simulink library "qss_tb_library_aalto"  (Simulink 8.3)
settings: Solver=ode45  SolverMode=SingleTasking  StartTime=0.0  StopTime=1220  RelTol=1e-3
undefined symbols (not defined in the file): c_BT_E1, c_BT_E2, c_BT_E3, c_BT_E4, c_BT_L1, c_BT_L2, c_BT_L3, c_BT_L4, cap_BT, cc_done, delta_h_C_air, DiscIntNeverNeededParam, dw_GG_c, eff_FC_max, eta_EG_map, eta_EM_map, g, h, H_o_m, H_u, I_BT_max, i_FC_in, i_FC_max, k1, k2, k3, k4, k_cs, M_air, manual_gearbox, P_CVT_opt, power_max, Q_BT_0, Q_BT_IC, Q_BT_min, Q_SC_IC, r_wheel, rchg_map_BT, rdis_map_BT, rho, rho_f, soc_map_BT, t_c, T_CE_max, T_EG_c, T_EG_max, T_EM_max, T_z, U_BT_0, V, V_CE_map, V_FC_out, voc_map_BT, w_CE_max, w_CE_upper, w_CVT_opt, w_EG_row, w_EG_upper, w_EM_row, w_EM_upper ... (+1)
libraries: simulink x4
(part 2 of 4)

== system qss_tb_library_aalto/Energy Buffer/Supercapacitor v2 ==
  P_SC : Inport
  Fcn : Fcn  Expr=(-u[2]/C_SC+sqrt(u[2]^2/C_SC^2-4*R_SC*u[1]))/(2*R_SC)
  Gain : Gain  Gain=1/C_SC  SaturateOnIntegerOverflow=on  OutDataTypeStr=Inherit: Same as input  ParamDataTypeStr=Inherit: Same as input
  Gain1 : Gain  Gain=h  SaturateOnIntegerOverflow=on  OutDataTypeStr=Inherit: Same as input  ParamDataTypeStr=Inherit: Same as input
  Mux : Mux  Inputs=2
  SC charge : UnitDelay  InitialCondition=Q_SC_IC  SampleTime=h
  Sum3 : Sum  SaturateOnIntegerOverflow=on  InputSameDT=on  OutDataTypeStr=Inherit: Same as first input
  Supervision supercap : Subsystem
  To Workspace1 : ToWorkspace  VariableName=I_SC  SampleTime=1
  To Workspace2 : ToWorkspace  VariableName=U_SC  SampleTime=1
  To Workspace3 : ToWorkspace  VariableName=Q_SC  SampleTime=1
  To Workspace4 : ToWorkspace  VariableName=P_SC  SampleTime=1
  U_SC : Outport  InitialOutput=0
  wires:
  Gain1/1 -> Sum3/1
  Mux/1 -> Fcn/1
  Sum3/1 -> SC charge/1
  SC charge/1 -> Sum3/2, Gain/1, Mux/2, Supervision supercap/1(Q_SC), To Workspace3/1
  Fcn/1 -> Gain1/1, To Workspace1/1
  Gain/1 -> U_SC/1, To Workspace2/1
  P_SC/1 -> To Workspace4/1, Mux/1, Supervision supercap/2(P_SC)

== system qss_tb_library_aalto/Energy Buffer/Supercapacitor v3 ==
  P_SC : Inport
  Fcn : Fcn  Expr=(-u[2]/C_SC+sqrt(u[2]^2/C_SC^2-4*R_SC*u[1]))/(2*R_SC)
  Gain : Gain  Gain=1/C_SC  SaturateOnIntegerOverflow=on  OutDataTypeStr=Inherit: Same as input  ParamDataTypeStr=Inherit: Same as input
  Gain1 : Gain  Gain=h  SaturateOnIntegerOverflow=on  OutDataTypeStr=Inherit: Same as input  ParamDataTypeStr=Inherit: Same as input
  Mux : Mux  Inputs=2
  SC charge : UnitDelay  InitialCondition=Q_SC_IC  SampleTime=h
  Sum3 : Sum  SaturateOnIntegerOverflow=on  InputSameDT=on  OutDataTypeStr=Inherit: Same as first input
  Supervision supercap : Subsystem
  To Workspace1 : ToWorkspace  VariableName=I_SC  SampleTime=1
  To Workspace2 : ToWorkspace  VariableName=U_SC  SampleTime=1
  To Workspace3 : ToWorkspace  VariableName=Q_SC  SampleTime=1
  To Workspace4 : ToWorkspace  VariableName=P_SC  SampleTime=1
  U_SC : Outport  InitialOutput=0
  wires:
  P_SC/1 -> Supervision supercap/2(P_SC), Mux/1, To Workspace4/1
  Gain/1 -> To Workspace2/1, U_SC/1
  Fcn/1 -> To Workspace1/1, Gain1/1
  SC charge/1 -> To Workspace3/1, Supervision supercap/1(Q_SC), Mux/2, Gain/1, Sum3/2
  Sum3/1 -> SC charge/1
  Mux/1 -> Fcn/1
  Gain1/1 -> Sum3/1

== system qss_tb_library_aalto/Energy Converter/Combustion Engine (Willans-approximation) ==
  w_gear : Inport
  dw_gear : Inport  Port=2
  T_gear : Inport  Port=3
  Constant1 : Constant  Value=P_aux
  Detect fuel cutoff : Subsystem
  Detect idle : Subsystem
  Engine efficiency : Subsystem
  Engine inertia : Gain  Gain=theta_CE  SaturateOnIntegerOverflow=on  OutDataTypeStr=Inherit: Same as input  ParamDataTypeStr=Inherit: Same as input
  Lower limit (fuel cutoff) : Saturate  UpperLimit=inf  LowerLimit=T_CE_cutoff
  Lower limit (speed at idle) : Saturate  UpperLimit=inf  LowerLimit=w_CE_idle
  Product : Product  Inputs=**/  SaturateOnIntegerOverflow=on  RndMeth=Zero  InputSameDT=on  OutDataTypeStr=Inherit: Same as first input
  To Workspace3 : ToWorkspace  VariableName=T_CE  SampleTime=-1
  To Workspace4 : ToWorkspace  VariableName=w_CE  SampleTime=-1
  To Workspace5 : ToWorkspace  VariableName=P_CE  SampleTime=-1
  Total power : Sum  SaturateOnIntegerOverflow=on  InputSameDT=on  OutDataTypeStr=Inherit: Same as first input
  Total torque : Sum  SaturateOnIntegerOverflow=on  InputSameDT=on  OutDataTypeStr=Inherit: Same as first input
  P_CE : Outport  InitialOutput=0
  wires:
  Engine efficiency/1(eta_CE) -> Product/3
  T_gear/1 -> Total torque/1
  dw_gear/1 -> Engine inertia/1
  Total torque/1 -> Lower limit (fuel cutoff)/1
  Engine inertia/1 -> Total torque/2
  Lower limit (fuel cutoff)/1 -> Detect idle/3(T_CE), Detect fuel cutoff/2(T_CE), Engine efficiency/2(T_CE), Product/2, To Workspace3/1
  Lower limit (speed at idle)/1 -> To Workspace4/1, Engine efficiency/1(w_CE), Detect idle/2(w_CE), Product/1
  w_gear/1 -> Lower limit (speed at idle)/1
  Product/1 -> Detect idle/1(P_CE_fuel)
  Detect idle/1(P_CE) -> Detect fuel cutoff/1(P_CE_fuel)
  Detect fuel cutoff/1(P_CE) -> Total power/1
  Total power/1 -> P_CE/1, To Workspace5/1
  Constant1/1 -> Total power/2

== system qss_tb_library_aalto/Energy Converter/Combustion Engine (consumption map) ==
  w_gear : Inport
  dw_gear : Inport  Port=2
  T_gear : Inport  Port=3
  Constant1 : Constant  Value=P_aux
  Detect fuel cutoff : Subsystem
  Detect idle : Subsystem
  Detect overload and overspeed : Subsystem
  "Engine consumption map V = f(w, T) [kg/s]" : Lookup2D  RowIndex=w_CE_row  ColumnIndex=T_CE_col  Table=V_CE_map
  Engine inertia : Gain  Gain=theta_CE  SaturateOnIntegerOverflow=on  OutDataTypeStr=Inherit: Same as input  ParamDataTypeStr=Inherit: Same as input
  Fuel lower heating value : Gain  Gain=H_u  SaturateOnIntegerOverflow=on  OutDataTypeStr=Inherit: Same as input  ParamDataTypeStr=Inherit: Same as input
  Lower limit (fuel cutoff) : Saturate  UpperLimit=inf  LowerLimit=T_CE_cutoff
  Lower limit (speed at idle) : Saturate  UpperLimit=inf  LowerLimit=w_CE_idle
  To Workspace3 : ToWorkspace  VariableName=T_CE  SampleTime=-1
  To Workspace4 : ToWorkspace  VariableName=w_CE  SampleTime=-1
  To Workspace5 : ToWorkspace  VariableName=P_CE  SampleTime=-1
  Total power : Sum  SaturateOnIntegerOverflow=on  InputSameDT=on  OutDataTypeStr=Inherit: Same as first input
  Total torque : Sum  SaturateOnIntegerOverflow=on  InputSameDT=on  OutDataTypeStr=Inherit: Same as first input
  P_CE : Outport  InitialOutput=0
  wires:
  T_gear/1 -> Total torque/1
  dw_gear/1 -> Engine inertia/1
  Total torque/1 -> Lower limit (fuel cutoff)/1
  Engine inertia/1 -> Total torque/2
  Lower limit (speed at idle)/1 -> Detect overload and overspeed/1(w_CE), Detect idle/2(w_CE), "Engine consumption map V = f(w, T) [kg/s]"/1, To Workspace4/1
  w_gear/1 -> Lower limit (speed at idle)/1
  Fuel lower heating value/1 -> Detect idle/1(P_CE_fuel)
  Detect idle/1(P_CE) -> Detect fuel cutoff/1(P_CE_fuel)
  "Engine consumption map V = f(w, T) [kg/s]"/1 -> Fuel lower heating value/1
  Detect fuel cutoff/1(P_CE) -> Total power/1
  Total power/1 -> P_CE/1, To Workspace5/1
  Constant1/1 -> Total power/2
  Lower limit (fuel cutoff)/1 -> Detect overload and overspeed/2(T_CE), "Engine consumption map V = f(w, T) [kg/s]"/2, Detect idle/3(T_CE), Detect fuel cutoff/2(T_CE), To Workspace3/1

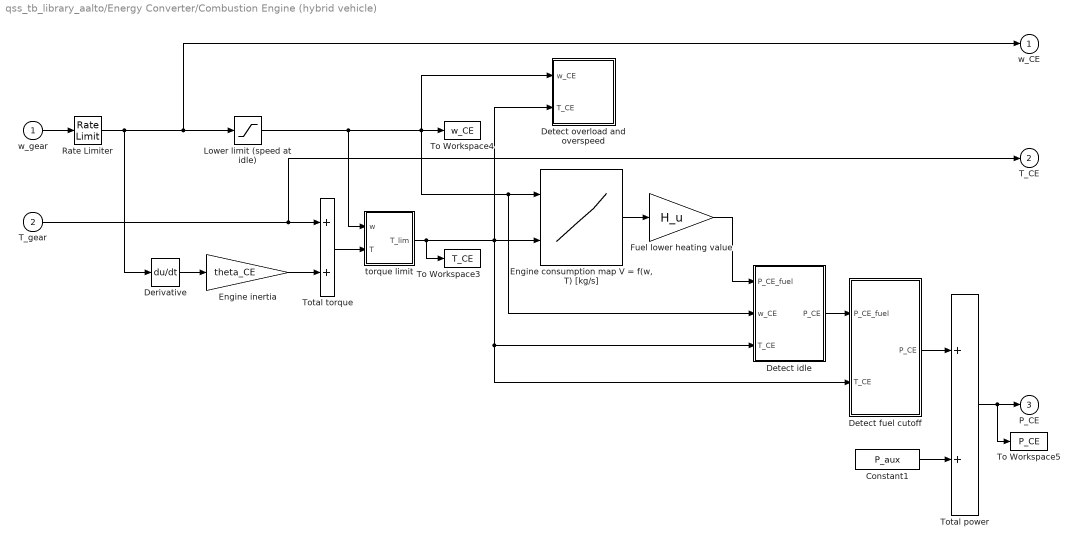
== system qss_tb_library_aalto/Energy Converter/Combustion Engine (hybrid vehicle) ==
  w_gear : Inport
  T_gear : Inport  Port=2
  Constant1 : Constant  Value=P_aux
  Derivative : Derivative
  Detect fuel cutoff : Subsystem
  Detect idle : Subsystem
  Detect overload and overspeed : Subsystem
  "Engine consumption map V = f(w, T) [kg/s]" : Lookup2D  RowIndex=w_CE_row  ColumnIndex=T_CE_col  Table=V_CE_map
  Engine inertia : Gain  Gain=theta_CE  SaturateOnIntegerOverflow=on  OutDataTypeStr=Inherit: Same as input  ParamDataTypeStr=Inherit: Same as input
  Fuel lower heating value : Gain  Gain=H_u  SaturateOnIntegerOverflow=on  OutDataTypeStr=Inherit: Same as input  ParamDataTypeStr=Inherit: Same as input
  Lower limit (speed at idle) : Saturate  UpperLimit=inf  LowerLimit=w_CE_idle*0
  Rate Limiter : RateLimiter  RisingSlewLimit=100  FallingSlewLimit=-250
  To Workspace3 : ToWorkspace  VariableName=T_CE  SampleTime=-1
  To Workspace4 : ToWorkspace  VariableName=w_CE  SampleTime=-1
  To Workspace5 : ToWorkspace  VariableName=P_CE  SampleTime=-1
  Total power : Sum  SaturateOnIntegerOverflow=on  InputSameDT=on  OutDataTypeStr=Inherit: Same as first input
  Total torque : Sum  SaturateOnIntegerOverflow=on  InputSameDT=on  OutDataTypeStr=Inherit: Same as first input
  torque limit : Subsystem
  w_CE : Outport  InitialOutput=0
  T_CE : Outport  Port=2  InitialOutput=0
  P_CE : Outport  Port=3  InitialOutput=0
  wires:
  torque limit/1(T_lim) -> To Workspace3/1, Detect fuel cutoff/2(T_CE), Detect idle/3(T_CE), "Engine consumption map V = f(w, T) [kg/s]"/2, Detect overload and overspeed/2(T_CE)
  Constant1/1 -> Total power/2
  Total power/1 -> To Workspace5/1, P_CE/1
  Detect fuel cutoff/1(P_CE) -> Total power/1
  "Engine consumption map V = f(w, T) [kg/s]"/1 -> Fuel lower heating value/1
  Detect idle/1(P_CE) -> Detect fuel cutoff/1(P_CE_fuel)
  Fuel lower heating value/1 -> Detect idle/1(P_CE_fuel)
  w_gear/1 -> Rate Limiter/1
  Engine inertia/1 -> Total torque/2
  T_gear/1 -> Total torque/1, T_CE/1
  Lower limit (speed at idle)/1 -> torque limit/1(w), Detect overload and overspeed/1(w_CE), To Workspace4/1, "Engine consumption map V = f(w, T) [kg/s]"/1, Detect idle/2(w_CE)
  Rate Limiter/1 -> Derivative/1, Lower limit (speed at idle)/1, w_CE/1
  Derivative/1 -> Engine inertia/1
  Total torque/1 -> torque limit/2(T)

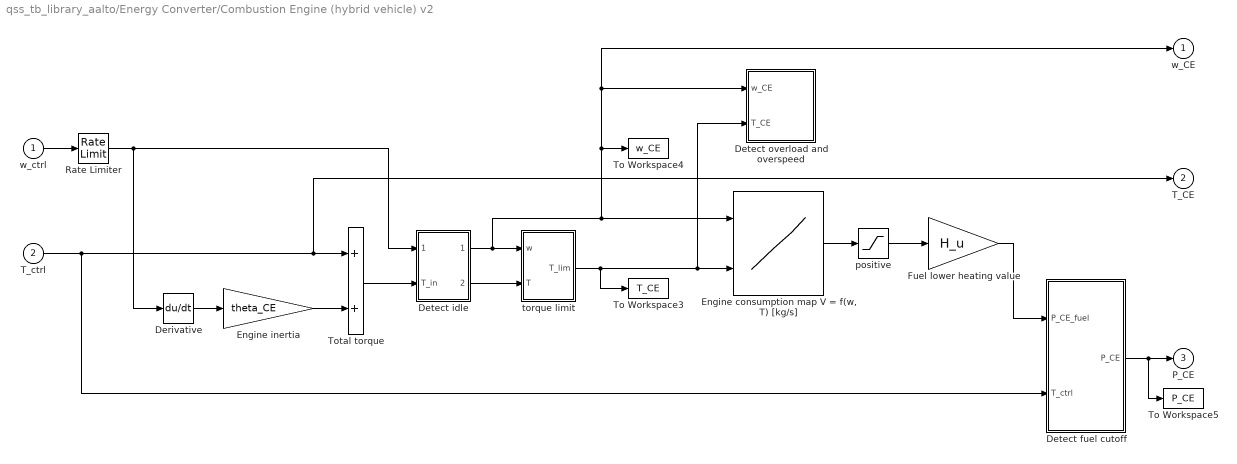
== system qss_tb_library_aalto/Energy Converter/Combustion Engine (hybrid vehicle) v2 ==
  w_ctrl : Inport
  T_ctrl : Inport  Port=2
  Derivative : Derivative
  Detect fuel cutoff : Subsystem
  Detect idle : Subsystem
  Detect overload and overspeed : Subsystem
  "Engine consumption map V = f(w, T) [kg/s]" : Lookup2D  RowIndex=w_CE_row  ColumnIndex=T_CE_col  Table=V_CE_map
  Engine inertia : Gain  Gain=theta_CE  SaturateOnIntegerOverflow=on  OutDataTypeStr=Inherit: Same as input  ParamDataTypeStr=Inherit: Same as input
  Fuel lower heating value : Gain  Gain=H_u  SaturateOnIntegerOverflow=on  OutDataTypeStr=Inherit: Same as input  ParamDataTypeStr=Inherit: Same as input
  Rate Limiter : RateLimiter  RisingSlewLimit=100  FallingSlewLimit=-250
  To Workspace3 : ToWorkspace  VariableName=T_CE  SampleTime=-1
  To Workspace4 : ToWorkspace  VariableName=w_CE  SampleTime=-1
  To Workspace5 : ToWorkspace  VariableName=P_CE  SampleTime=-1
  Total torque : Sum  SaturateOnIntegerOverflow=on  InputSameDT=on  OutDataTypeStr=Inherit: Same as first input
  "positive " : Saturate  UpperLimit=inf  LowerLimit=0
  torque limit : Subsystem
  w_CE : Outport  InitialOutput=0
  T_CE : Outport  Port=2  InitialOutput=0
  P_CE : Outport  Port=3  InitialOutput=0
  wires:
  Total torque/1 -> Detect idle/2(T_in)
  Derivative/1 -> Engine inertia/1
  Rate Limiter/1 -> Detect idle/1(w_CE), Derivative/1
  T_ctrl/1 -> Detect fuel cutoff/2(T_ctrl), T_CE/1, Total torque/1
  Engine inertia/1 -> Total torque/2
  w_ctrl/1 -> Rate Limiter/1
  Fuel lower heating value/1 -> Detect fuel cutoff/1(P_CE_fuel)
  "Engine consumption map V = f(w, T) [kg/s]"/1 -> "positive "/1
  Detect fuel cutoff/1(P_CE) -> P_CE/1, To Workspace5/1
  torque limit/1(T_lim) -> To Workspace3/1, Detect overload and overspeed/2(T_CE), "Engine consumption map V = f(w, T) [kg/s]"/2
  "positive "/1 -> Fuel lower heating value/1
  Detect idle/2(T_out) -> torque limit/2(T)
  Detect idle/1(w_out) -> w_CE/1, Detect overload and overspeed/1(w_CE), To Workspace4/1, "Engine consumption map V = f(w, T) [kg/s]"/1, torque limit/1(w)

== system qss_tb_library_aalto/Energy Converter/Combustion Engine v2 ==
  w_gear : Inport
  dw_gear : Inport  Port=2
  T_gear : Inport  Port=3
  Constant1 : Constant  Value=P_aux
  Detect fuel cutoff : Subsystem
  Detect idle : Subsystem
  Detect overload and overspeed : Subsystem
  "Engine consumption map V = f(w, T) [kg/s]" : Lookup2D  RowIndex=w_CE_row  ColumnIndex=T_CE_col  Table=V_CE_map
  Engine inertia : Gain  Gain=theta_CE  SaturateOnIntegerOverflow=on  OutDataTypeStr=Inherit: Same as input  ParamDataTypeStr=Inherit: Same as input
  Fuel lower heating value : Gain  Gain=H_u  SaturateOnIntegerOverflow=on  OutDataTypeStr=Inherit: Same as input  ParamDataTypeStr=Inherit: Same as input
  Lower limit (fuel cutoff) : Saturate  UpperLimit=inf  LowerLimit=T_CE_cutoff
  Lower limit (speed at idle) : Saturate  UpperLimit=inf  LowerLimit=w_CE_idle
  To Workspace3 : ToWorkspace  VariableName=T_CE  SampleTime=-1
  To Workspace4 : ToWorkspace  VariableName=w_CE  SampleTime=-1
  To Workspace5 : ToWorkspace  VariableName=P_CE  SampleTime=-1
  Total power : Sum  SaturateOnIntegerOverflow=on  InputSameDT=on  OutDataTypeStr=Inherit: Same as first input
  Total torque : Sum  SaturateOnIntegerOverflow=on  InputSameDT=on  OutDataTypeStr=Inherit: Same as first input
  P_CE : Outport  InitialOutput=0
  wires:
  Lower limit (fuel cutoff)/1 -> To Workspace3/1, Detect fuel cutoff/2(T_CE), Detect idle/3(T_CE), "Engine consumption map V = f(w, T) [kg/s]"/2, Detect overload and overspeed/2(T_CE)
  Constant1/1 -> Total power/2
  Total power/1 -> To Workspace5/1, P_CE/1
  Detect fuel cutoff/1(P_CE) -> Total power/1
  "Engine consumption map V = f(w, T) [kg/s]"/1 -> Fuel lower heating value/1
  Detect idle/1(P_CE) -> Detect fuel cutoff/1(P_CE_fuel)
  Fuel lower heating value/1 -> Detect idle/1(P_CE_fuel)
  w_gear/1 -> Lower limit (speed at idle)/1
  Lower limit (speed at idle)/1 -> To Workspace4/1, "Engine consumption map V = f(w, T) [kg/s]"/1, Detect idle/2(w_CE), Detect overload and overspeed/1(w_CE)
  Engine inertia/1 -> Total torque/2
  Total torque/1 -> Lower limit (fuel cutoff)/1
  dw_gear/1 -> Engine inertia/1
  T_gear/1 -> Total torque/1

== system qss_tb_library_aalto/Energy Converter/Combustion Engine v3 ==
  w_gear : Inport
  dw_gear : Inport  Port=2
  T_gear : Inport  Port=3
  Detect fuel cutoff : Subsystem
  Detect idle : Subsystem
  Detect overload and overspeed : Subsystem
  "Engine consumption map V = f(w, T) [kg/s]" : Lookup2D  RowIndex=w_CE_row  ColumnIndex=T_CE_col  Table=V_CE_map
  Engine inertia : Gain  Gain=theta_CE  SaturateOnIntegerOverflow=on  OutDataTypeStr=Inherit: Same as input  ParamDataTypeStr=Inherit: Same as input
  Fuel lower heating value : Gain  Gain=H_u  SaturateOnIntegerOverflow=on  OutDataTypeStr=Inherit: Same as input  ParamDataTypeStr=Inherit: Same as input
  Lower limit (fuel cutoff) : Saturate  UpperLimit=inf  LowerLimit=T_CE_cutoff
  Lower limit (speed at idle) : Saturate  UpperLimit=inf  LowerLimit=w_CE_idle
  To Workspace3 : ToWorkspace  VariableName=T_CE  SampleTime=-1
  To Workspace4 : ToWorkspace  VariableName=w_CE  SampleTime=-1
  To Workspace5 : ToWorkspace  VariableName=P_CE  SampleTime=-1
  Total torque : Sum  SaturateOnIntegerOverflow=on  InputSameDT=on  OutDataTypeStr=Inherit: Same as first input
  P_CE : Outport  InitialOutput=0
  wires:
  T_gear/1 -> Detect fuel cutoff/2(T_gear), Total torque/1
  dw_gear/1 -> Engine inertia/1
  Engine inertia/1 -> Total torque/2
  Lower limit (speed at idle)/1 -> Detect overload and overspeed/1(w_CE), "Engine consumption map V = f(w, T) [kg/s]"/1, To Workspace4/1, Detect idle/1(w_CE)
  w_gear/1 -> Lower limit (speed at idle)/1
  "Engine consumption map V = f(w, T) [kg/s]"/1 -> Fuel lower heating value/1
  Detect idle/1(T_out) -> Lower limit (fuel cutoff)/1
  Lower limit (fuel cutoff)/1 -> Detect overload and overspeed/2(T_CE), "Engine consumption map V = f(w, T) [kg/s]"/2, To Workspace3/1
  Total torque/1 -> Detect idle/2(T_in)
  Fuel lower heating value/1 -> Detect fuel cutoff/1(P_CE_fuel)
  Detect fuel cutoff/1(P_CE) -> To Workspace5/1, P_CE/1

== system qss_tb_library_aalto/Energy Converter/Electric Generator ==
  w_gear : Inport
  T_gear : Inport  Port=2
  Detect overload and overspeed : Subsystem
  "Efficiency eta = f(w, T)" : Lookup2D  RowIndex=w_EG_row  ColumnIndex=T_EG_col  Table=eta_EG_map
  Product : Product  Inputs=3  SaturateOnIntegerOverflow=on  RndMeth=Zero  InputSameDT=on  OutDataTypeStr=Inherit: Same as first input
  To Workspace1 : ToWorkspace  VariableName=w_EG  SampleTime=-1
  To Workspace2 : ToWorkspace  VariableName=T_EG  SampleTime=-1
  To Workspace5 : ToWorkspace  VariableName=P_EG  SampleTime=-1
  P_EG : Outport  InitialOutput=0
  wires:
  T_gear/1 -> Product/2, "Efficiency eta = f(w, T)"/2, Detect overload and overspeed/2(T_EG), To Workspace2/1
  "Efficiency eta = f(w, T)"/1 -> Product/1
  Product/1 -> P_EG/1, To Workspace5/1
  w_gear/1 -> Product/3, "Efficiency eta = f(w, T)"/1, Detect overload and overspeed/1(w_EG), To Workspace1/1

== system qss_tb_library_aalto/Energy Converter/Electric Generator v2 ==
  w_gear : Inport
  T_gear : Inport  Port=2
  Detect overload and overspeed : Subsystem
  "Efficiency eta = f(w, T)" : Lookup2D  RowIndex=w_EG_row  ColumnIndex=T_EG_col  Table=eta_EG_map
  Product : Product  Inputs=3  SaturateOnIntegerOverflow=on  RndMeth=Zero  InputSameDT=on  OutDataTypeStr=Inherit: Same as first input
  To Workspace1 : ToWorkspace  VariableName=w_EG  SampleTime=-1
  To Workspace2 : ToWorkspace  VariableName=T_EG  SampleTime=-1
  To Workspace5 : ToWorkspace  VariableName=P_EG  SampleTime=-1
  P_EG : Outport  InitialOutput=0
  wires:
  w_gear/1 -> To Workspace1/1, Detect overload and overspeed/1(w_EG), "Efficiency eta = f(w, T)"/1, Product/3
  Product/1 -> To Workspace5/1, P_EG/1
  "Efficiency eta = f(w, T)"/1 -> Product/1
  T_gear/1 -> To Workspace2/1, Detect overload and overspeed/2(T_EG), "Efficiency eta = f(w, T)"/2, Product/2

== system qss_tb_library_aalto/Energy Converter/Electric Generator v3 ==
  w_gear : Inport
  T_gear : Inport  Port=2
  Detect overload and overspeed : Subsystem
  "Efficiency eta = f(w, T)" : Lookup2D  RowIndex=w_EG_row  ColumnIndex=T_EG_col  Table=eta_EG_map
  Product : Product  Inputs=3  SaturateOnIntegerOverflow=on  RndMeth=Zero  InputSameDT=on  OutDataTypeStr=Inherit: Same as first input
  Switch1 : Switch  Criteria=u2 > Threshold  SaturateOnIntegerOverflow=on  InputSameDT=on
  To Workspace1 : ToWorkspace  VariableName=w_EG  SampleTime=-1
  To Workspace2 : ToWorkspace  VariableName=T_EG  SampleTime=-1
  To Workspace5 : ToWorkspace  VariableName=P_EG  SampleTime=-1
  inverse : Fcn  Expr=1/u(1)
  P_EG : Outport  InitialOutput=0
  wires:
  w_gear/1 -> To Workspace1/1, Detect overload and overspeed/1(w_EG), "Efficiency eta = f(w, T)"/1, Product/3
  Product/1 -> To Workspace5/1, P_EG/1
  "Efficiency eta = f(w, T)"/1 -> inverse/1, Switch1/1
  T_gear/1 -> To Workspace2/1, Detect overload and overspeed/2(T_EG), "Efficiency eta = f(w, T)"/2, Switch1/2, Product/2
  Switch1/1 -> Product/1
  inverse/1 -> Switch1/3

== system qss_tb_library_aalto/Energy Converter/Electric Motor ==
  w_gear : Inport
  dw_gear : Inport  Port=2
  T_gear : Inport  Port=3
  Constant1 : Constant  Value=P_aux
  Detect overload and overspeed : Subsystem
  "Efficiency eta = f(w, T)" : Lookup2D  RowIndex=w_EM_row  ColumnIndex=T_EM_col  Table=eta_EM_map
  Gain1 : Gain  Gain=theta_EM  SaturateOnIntegerOverflow=on  OutDataTypeStr=Inherit: Same as input  ParamDataTypeStr=Inherit: Same as input
  Product : Product  Inputs=3  SaturateOnIntegerOverflow=on  RndMeth=Zero  InputSameDT=on  OutDataTypeStr=Inherit: Same as first input
  To Workspace1 : ToWorkspace  VariableName=w_EM  SampleTime=-1
  To Workspace2 : ToWorkspace  VariableName=T_EM  SampleTime=-1
  To Workspace5 : ToWorkspace  VariableName=P_EM  SampleTime=-1
  Total power : Sum  SaturateOnIntegerOverflow=on  InputSameDT=on  OutDataTypeStr=Inherit: Same as first input
  Total torque : Sum  SaturateOnIntegerOverflow=on  InputSameDT=on  OutDataTypeStr=Inherit: Same as first input
  P_EM : Outport  InitialOutput=0
  wires:
  w_gear/1 -> Detect overload and overspeed/1(w_EM), "Efficiency eta = f(w, T)"/1, Product/3, To Workspace1/1
  "Efficiency eta = f(w, T)"/1 -> Product/1
  dw_gear/1 -> Gain1/1
  T_gear/1 -> Total torque/2
  Gain1/1 -> Total torque/1
  Total torque/1 -> Detect overload and overspeed/2(T_EM), "Efficiency eta = f(w, T)"/2, Product/2, To Workspace2/1
  Constant1/1 -> Total power/2
  Product/1 -> Total power/1
  Total power/1 -> P_EM/1, To Workspace5/1

== system qss_tb_library_aalto/Energy Converter/Electric Motor v2 ==
  w_gear : Inport
  dw_gear : Inport  Port=2
  T_gear : Inport  Port=3
  Constant1 : Constant  Value=P_aux
  Detect overload and overspeed : Subsystem
  "Efficiency eta = f(w, T)" : Lookup2D  RowIndex=w_EM_row  ColumnIndex=T_EM_col  Table=eta_EM_map
  Gain1 : Gain  Gain=theta_EM  SaturateOnIntegerOverflow=on  OutDataTypeStr=Inherit: Same as input  ParamDataTypeStr=Inherit: Same as input
  Product : Product  Inputs=3  SaturateOnIntegerOverflow=on  RndMeth=Zero  InputSameDT=on  OutDataTypeStr=Inherit: Same as first input
  To Workspace1 : ToWorkspace  VariableName=w_EM  SampleTime=-1
  To Workspace2 : ToWorkspace  VariableName=T_EM  SampleTime=-1
  To Workspace5 : ToWorkspace  VariableName=P_EM  SampleTime=-1
  Total power : Sum  SaturateOnIntegerOverflow=on  InputSameDT=on  OutDataTypeStr=Inherit: Same as first input
  Total torque : Sum  SaturateOnIntegerOverflow=on  InputSameDT=on  OutDataTypeStr=Inherit: Same as first input
  P_EM : Outport  InitialOutput=0
  wires:
  Total power/1 -> To Workspace5/1, P_EM/1
  Product/1 -> Total power/1
  Constant1/1 -> Total power/2
  Total torque/1 -> To Workspace2/1, Product/2, "Efficiency eta = f(w, T)"/2, Detect overload and overspeed/2(T_EM)
  Gain1/1 -> Total torque/1
  T_gear/1 -> Total torque/2
  dw_gear/1 -> Gain1/1
  "Efficiency eta = f(w, T)"/1 -> Product/1
  w_gear/1 -> To Workspace1/1, Product/3, "Efficiency eta = f(w, T)"/1, Detect overload and overspeed/1(w_EM)

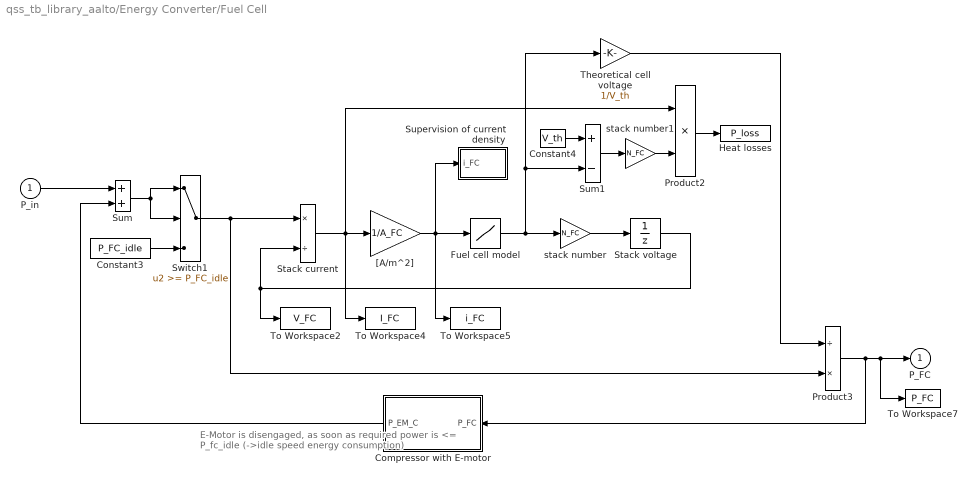
== system qss_tb_library_aalto/Energy Converter/Fuel Cell ==
  note: E-Motor is disengaged, as soon as required power
      |  is <= P_fc_idle (->idle speed energy consumption)
  P_in : Inport
  Compressor with E-motor : Subsystem
  Constant3 : Constant  Value=P_FC_idle
  Constant4 : Constant  Value=V_th
  Fuel cell model : Lookup  InputValues=i_FC_in  Table=V_FC_out  SaturateOnIntegerOverflow=on
  Heat losses : ToWorkspace  VariableName=P_loss  SampleTime=1
  Product2 : Product  SaturateOnIntegerOverflow=on  RndMeth=Zero  InputSameDT=on  OutDataTypeStr=Inherit: Same as first input
  Product3 : Product  Inputs=/*  SaturateOnIntegerOverflow=on  RndMeth=Zero  InputSameDT=on  OutDataTypeStr=Inherit: Same as first input
  Stack current : Product  Inputs=*/  SaturateOnIntegerOverflow=on  RndMeth=Zero  InputSameDT=on  OutDataTypeStr=Inherit: Same as first input
  Stack voltage : UnitDelay  InitialCondition=10  SampleTime=h
  Sum : Sum  SaturateOnIntegerOverflow=on  InputSameDT=on  OutDataTypeStr=Inherit: Same as first input
  Sum1 : Sum  Inputs=+-  SaturateOnIntegerOverflow=on  InputSameDT=on  OutDataTypeStr=Inherit: Same as first input
  Supervision of current density : Subsystem
  Switch1 : Switch  Threshold=P_FC_idle  SaturateOnIntegerOverflow=on  InputSameDT=on
  Theoretical cell voltage : Gain  Gain=1/V_th  SaturateOnIntegerOverflow=on  OutDataTypeStr=Inherit: Same as input  ParamDataTypeStr=Inherit: Same as input
  To Workspace2 : ToWorkspace  VariableName=V_FC  SampleTime=1
  To Workspace4 : ToWorkspace  VariableName=I_FC  SampleTime=1
  To Workspace5 : ToWorkspace  VariableName=i_FC  SampleTime=1
  To Workspace7 : ToWorkspace  VariableName=P_FC  SampleTime=1
  "[A/m^2]" : Gain  Gain=1/A_FC  SaturateOnIntegerOverflow=on  OutDataTypeStr=Inherit: Same as input  ParamDataTypeStr=Inherit: Same as input
  stack number : Gain  Gain=N_FC  SaturateOnIntegerOverflow=on  OutDataTypeStr=Inherit: Same as input  ParamDataTypeStr=Inherit: Same as input
  stack number1 : Gain  Gain=N_FC  SaturateOnIntegerOverflow=on  OutDataTypeStr=Inherit: Same as input  ParamDataTypeStr=Inherit: Same as input
  P_FC : Outport  InitialOutput=0
  wires:
  Compressor with E-motor/1(P_EM_C) -> Sum/2
  Switch1/1 -> Stack current/1, Product3/2
  Constant3/1 -> Switch1/3
  Sum/1 -> Switch1/2, Switch1/1
  P_in/1 -> Sum/1
  Constant4/1 -> Sum1/1
  stack number/1 -> Stack voltage/1
  Sum1/1 -> stack number1/1
  stack number1/1 -> Product2/2
  "[A/m^2]"/1 -> Fuel cell model/1, To Workspace5/1, Supervision of current density/1("   i_FC")
  Theoretical cell voltage/1 -> Product3/1
  Fuel cell model/1 -> stack number/1, Sum1/2, Theoretical cell voltage/1
  Stack current/1 -> "[A/m^2]"/1, Product2/1, To Workspace4/1
  Stack voltage/1 -> Stack current/2, To Workspace2/1
  Product3/1 -> P_FC/1, To Workspace7/1, Compressor with E-motor/1(P_FC)
  Product2/1 -> Heat losses/1

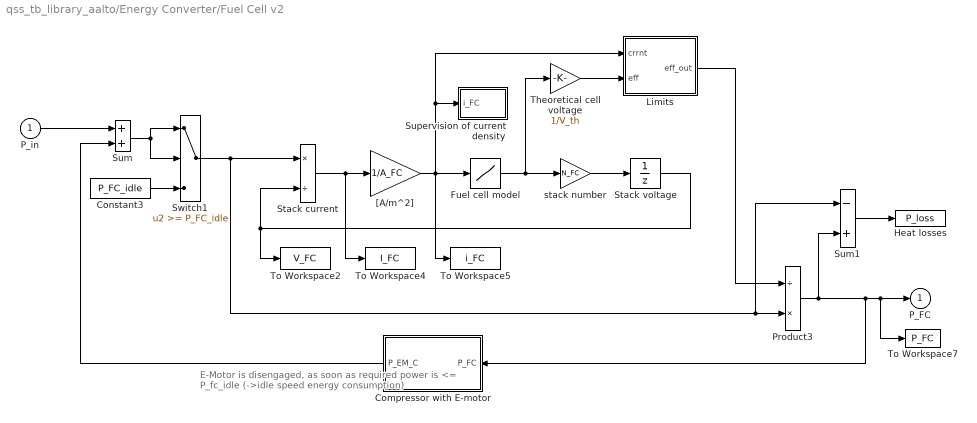
== system qss_tb_library_aalto/Energy Converter/Fuel Cell v2 ==
  note: E-Motor is disengaged, as soon as required power
      |  is <= P_fc_idle (->idle speed energy consumption)
  P_in : Inport
  Compressor with E-motor : Subsystem
  Constant3 : Constant  Value=P_FC_idle
  Fuel cell model : Lookup  InputValues=i_FC_in  Table=V_FC_out  SaturateOnIntegerOverflow=on
  Heat losses : ToWorkspace  VariableName=P_loss  SampleTime=1
  Limits : Subsystem
  Product3 : Product  Inputs=/*  SaturateOnIntegerOverflow=on  RndMeth=Zero  InputSameDT=on  OutDataTypeStr=Inherit: Same as first input
  Stack current : Product  Inputs=*/  SaturateOnIntegerOverflow=on  RndMeth=Zero  InputSameDT=on  OutDataTypeStr=Inherit: Same as first input
  Stack voltage : UnitDelay  InitialCondition=10  SampleTime=h
  Sum : Sum  SaturateOnIntegerOverflow=on  InputSameDT=on  OutDataTypeStr=Inherit: Same as first input
  Sum1 : Sum  Inputs=-+  SaturateOnIntegerOverflow=on  InputSameDT=on  OutDataTypeStr=Inherit: Same as first input
  Supervision of current density : Subsystem
  Switch1 : Switch  Threshold=P_FC_idle  SaturateOnIntegerOverflow=on  InputSameDT=on
  Theoretical cell voltage : Gain  Gain=1/V_th  SaturateOnIntegerOverflow=on  OutDataTypeStr=Inherit: Same as input  ParamDataTypeStr=Inherit: Same as input
  To Workspace2 : ToWorkspace  VariableName=V_FC  SampleTime=1
  To Workspace4 : ToWorkspace  VariableName=I_FC  SampleTime=1
  To Workspace5 : ToWorkspace  VariableName=i_FC  SampleTime=1
  To Workspace7 : ToWorkspace  VariableName=P_FC  SampleTime=1
  "[A/m^2]" : Gain  Gain=1/A_FC  SaturateOnIntegerOverflow=on  OutDataTypeStr=Inherit: Same as input  ParamDataTypeStr=Inherit: Same as input
  stack number : Gain  Gain=N_FC  SaturateOnIntegerOverflow=on  OutDataTypeStr=Inherit: Same as input  ParamDataTypeStr=Inherit: Same as input
  P_FC : Outport  InitialOutput=0
  wires:
  Compressor with E-motor/1(P_EM_C) -> Sum/2
  Switch1/1 -> Stack current/1, Sum1/1, Product3/2
  Constant3/1 -> Switch1/3
  Sum/1 -> Switch1/2, Switch1/1
  P_in/1 -> Sum/1
  stack number/1 -> Stack voltage/1
  "[A/m^2]"/1 -> Fuel cell model/1, To Workspace5/1, Limits/1(crrnt), Supervision of current density/1("   i_FC")
  Fuel cell model/1 -> stack number/1, Theoretical cell voltage/1
  Stack current/1 -> "[A/m^2]"/1, To Workspace4/1
  Stack voltage/1 -> Stack current/2, To Workspace2/1
  Product3/1 -> Sum1/2, P_FC/1, To Workspace7/1, Compressor with E-motor/1(P_FC)
  Theoretical cell voltage/1 -> Limits/2(eff)
  Limits/1(eff_out) -> Product3/1
  Sum1/1 -> Heat losses/1

== system qss_tb_library_aalto/Energy Source/Hydrogen Tank ==
  P_fuel : Inport
  x_tot : Inport  Port=2
  Fu2131el density1 : Gain  Gain=1/0.745  SaturateOnIntegerOverflow=on  OutDataTypeStr=Inherit: Same as input  ParamDataTypeStr=Inherit: Same as input
  Gain1 : Gain  Gain=1e5  SaturateOnIntegerOverflow=on  OutDataTypeStr=Inherit: Same as input  ParamDataTypeStr=Inherit: Same as input
  Gain3 : Gain  Gain=1e5  SaturateOnIntegerOverflow=on  OutDataTypeStr=Inherit: Same as input  ParamDataTypeStr=Inherit: Same as input
  Integration : Subsystem
  Product : Product  Inputs=*/  SaturateOnIntegerOverflow=on  RndMeth=Zero  InputSameDT=on  OutDataTypeStr=Inherit: Same as first input
  Product1 : Product  Inputs=/*  SaturateOnIntegerOverflow=on  RndMeth=Zero  InputSameDT=on  OutDataTypeStr=Inherit: Same as first input
  To Workspace7 : ToWorkspace  VariableName=M_kg  SampleTime=-1
  kg/100 km : Outport  InitialOutput=0
  liter/100 km : Outport  Port=2  InitialOutput=0
  wires:
  Product/1 -> Gain3/1
  Integration/1(m_fuel) -> Product/1
  Gain3/1 -> To Workspace7/1, kg/100 km/1
  x_tot/1 -> Product1/1, Product/2
  P_fuel/1 -> Integration/1(P_fuel)
  Integration/2(gas equivalent) -> Fu2131el density1/1
  Fu2131el density1/1 -> Product1/2
  Product1/1 -> Gain1/1
  Gain1/1 -> liter/100 km/1

== system qss_tb_library_aalto/Energy Source/Tank ==
  P_fuel : Inport
  x_tot : Inport  Port=2
  Factor for cold start : Gain  Gain=k_cs  SaturateOnIntegerOverflow=on  OutDataTypeStr=Inherit: Same as input  ParamDataTypeStr=Inherit: Same as input
  Fu2131el density : Gain  Gain=1/rho_f  SaturateOnIntegerOverflow=on  OutDataTypeStr=Inherit: Same as input  ParamDataTypeStr=Inherit: Same as input
  Gain3 : Gain  Gain=1e5  SaturateOnIntegerOverflow=on  OutDataTypeStr=Inherit: Same as input  ParamDataTypeStr=Inherit: Same as input
  Integration : Subsystem
  Product : Product  Inputs=*/  SaturateOnIntegerOverflow=on  RndMeth=Zero  InputSameDT=on  OutDataTypeStr=Inherit: Same as first input
  To Workspace7 : ToWorkspace  VariableName=V_liter  SampleTime=-1
  liter/100 km : Outport  InitialOutput=0
  wires:
  P_fuel/1 -> Integration/1(P_fuel)
  x_tot/1 -> Product/2
  Integration/1(m_fuel) -> Fu2131el density/1
  Gain3/1 -> liter/100 km/1, To Workspace7/1
  Fu2131el density/1 -> Product/1
  Product/1 -> Factor for cold start/1
  Factor for cold start/1 -> Gain3/1

== system qss_tb_library_aalto/Energy Source/Tank v2 ==
  P_fuel : Inport
  x_tot : Inport  Port=2
  Fu2131el density : Gain  Gain=1/rho_f  SaturateOnIntegerOverflow=on  OutDataTypeStr=Inherit: Same as input  ParamDataTypeStr=Inherit: Same as input
  Gain3 : Gain  Gain=1e5  SaturateOnIntegerOverflow=on  OutDataTypeStr=Inherit: Same as input  ParamDataTypeStr=Inherit: Same as input
  Integration : Subsystem
  Product : Product  Inputs=*/  SaturateOnIntegerOverflow=on  RndMeth=Zero  InputSameDT=on  OutDataTypeStr=Inherit: Same as first input
  To Workspace7 : ToWorkspace  VariableName=V_liter  SampleTime=-1
  liter/100 km : Outport  InitialOutput=0
  wires:
  Product/1 -> Gain3/1
  Fu2131el density/1 -> Product/1
  Gain3/1 -> To Workspace7/1, liter/100 km/1
  Integration/1(m_fuel) -> Fu2131el density/1
  x_tot/1 -> Product/2
  P_fuel/1 -> Integration/1(P_fuel)

== system qss_tb_library_aalto/Gear System/Continuously Variable Transmission ==
  w_wheel : Inport
  dw_wheel : Inport  Port=2
  T_wheel : Inport  Port=3
  j_CVT : Inport  Port=4
  dj_CVT : Inport  Port=5
  Power flow : Subsystem
  Product{,1..3} (4 alike) : Product  SaturateOnIntegerOverflow=on  RndMeth=Zero  InputSameDT=on  OutDataTypeStr=Inherit: Same as first input
  Sum : Sum  SaturateOnIntegerOverflow=on  InputSameDT=on  OutDataTypeStr=Inherit: Same as first input
  To Workspace1 : ToWorkspace  VariableName=w_CVT  SampleTime=-1
  To Workspace8 : ToWorkspace  VariableName=P_CVT  SampleTime=-1
  To Workspace9 : ToWorkspace  VariableName=T_CVT  SampleTime=-1
  w_CVT : Outport  InitialOutput=0
  dw_CVT : Outport  Port=2  InitialOutput=0
  T_CVT : Outport  Port=3  InitialOutput=0
  wires:
  w_wheel/1 -> Power flow/1(w_wheel), Product2/1, Product/1
  Power flow/1(T_CVT) -> To Workspace9/1, T_CVT/1, Product3/2
  Product/1 -> Product3/1, w_CVT/1, To Workspace1/1
  Sum/1 -> dw_CVT/1
  dw_wheel/1 -> Product1/1
  dj_CVT/1 -> Product2/2
  j_CVT/1 -> Product1/2, Product/2, Power flow/3(j_CVT)
  Product1/1 -> Sum/2
  Product2/1 -> Sum/1
  T_wheel/1 -> Power flow/2(T_wheel)
  Product3/1 -> To Workspace8/1

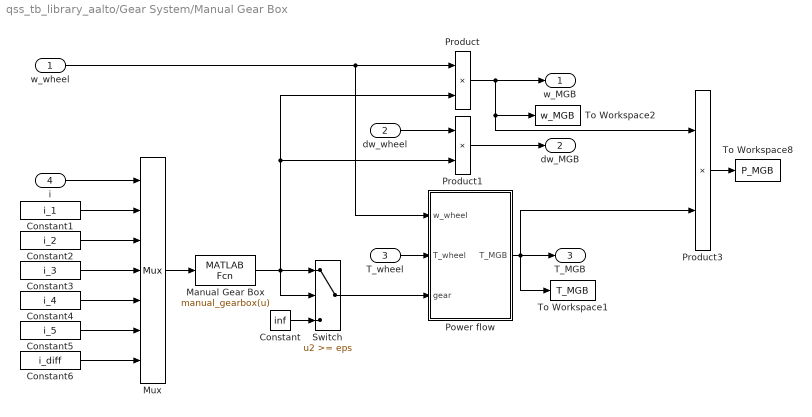
== system qss_tb_library_aalto/Gear System/Manual Gear Box ==
  w_wheel : Inport
  dw_wheel : Inport  Port=2
  T_wheel : Inport  Port=3
  i : Inport  Port=4
  Constant : Constant  Value=inf
  Constant1 : Constant  Value=i_1
  Constant2 : Constant  Value=i_2
  Constant3 : Constant  Value=i_3
  Constant4 : Constant  Value=i_4
  Constant5 : Constant  Value=i_5
  Constant6 : Constant  Value=i_diff
  Manual Gear Box : MATLABFcn  MATLABFcn=manual_gearbox(u)  OutputDimensions=1
  Mux : Mux  Inputs=7
  Power flow : Subsystem
  Product : Product  SaturateOnIntegerOverflow=on  RndMeth=Zero  InputSameDT=on  OutDataTypeStr=Inherit: Same as first input
  Product1 : Product  SaturateOnIntegerOverflow=on  RndMeth=Zero  InputSameDT=on  OutDataTypeStr=Inherit: Same as first input
  Product3 : Product  SaturateOnIntegerOverflow=on  RndMeth=Zero  InputSameDT=on  OutDataTypeStr=Inherit: Same as first input
  Switch : Switch  Threshold=eps  SaturateOnIntegerOverflow=on  InputSameDT=on
  To Workspace1 : ToWorkspace  VariableName=T_MGB  SampleTime=-1
  To Workspace2 : ToWorkspace  VariableName=w_MGB  SampleTime=-1
  To Workspace8 : ToWorkspace  VariableName=P_MGB  SampleTime=-1
  w_MGB : Outport  InitialOutput=0
  dw_MGB : Outport  Port=2  InitialOutput=0
  T_MGB : Outport  Port=3  InitialOutput=0
  wires:
  Power flow/1(T_MGB) -> T_MGB/1, Product3/2, To Workspace1/1
  Product/1 -> w_MGB/1, Product3/1, To Workspace2/1
  Constant/1 -> Switch/3
  w_wheel/1 -> Product/1, Power flow/1(w_wheel)
  Product1/1 -> dw_MGB/1
  dw_wheel/1 -> Product1/1
  Manual Gear Box/1 -> Product/2, Product1/2, Switch/2, Switch/1
  Product3/1 -> To Workspace8/1
  Switch/1 -> Power flow/3(gear)
  T_wheel/1 -> Power flow/2(T_wheel)
  Constant1/1 -> Mux/2
  Constant2/1 -> Mux/3
  Constant3/1 -> Mux/4
  Constant4/1 -> Mux/5
  Constant5/1 -> Mux/6
  Constant6/1 -> Mux/7
  i/1 -> Mux/1
  Mux/1 -> Manual Gear Box/1

== system qss_tb_library_aalto/Gear System/Simple Transmission ==
  w_wheel : Inport
  dw_wheel : Inport  Port=2
  T_wheel : Inport  Port=3
  Constant : Constant  Value=gear_ratio
  Power flow : Subsystem
  Product : Product  SaturateOnIntegerOverflow=on  RndMeth=Zero  InputSameDT=on  OutDataTypeStr=Inherit: Same as first input
  Product1 : Product  SaturateOnIntegerOverflow=on  RndMeth=Zero  InputSameDT=on  OutDataTypeStr=Inherit: Same as first input
  Product3 : Product  SaturateOnIntegerOverflow=on  RndMeth=Zero  InputSameDT=on  OutDataTypeStr=Inherit: Same as first input
  To Workspace1 : ToWorkspace  VariableName=w_trans  SampleTime=-1
  To Workspace2 : ToWorkspace  VariableName=T_trans  SampleTime=-1
  To Workspace3 : ToWorkspace  VariableName=P_trans  SampleTime=-1
  w_trans : Outport  InitialOutput=0
  dw_trans : Outport  Port=2  InitialOutput=0
  T_trans : Outport  Port=3  InitialOutput=0
  wires:
  Power flow/1(T_trans) -> T_trans/1, To Workspace2/1, Product3/2
  Product1/1 -> dw_trans/1
  Product/1 -> w_trans/1, To Workspace1/1, Product3/1
  dw_wheel/1 -> Product1/1
  T_wheel/1 -> Power flow/2(T_wheel)
  Constant/1 -> Power flow/3(gear_ratio), Product1/2, Product/2
  w_wheel/1 -> Product/1, Power flow/1(w_wheel)
  Product3/1 -> To Workspace3/1

== system qss_tb_library_aalto/Gear System/Transmission CE-EG ==
  w_wheel : Inport
  dw_wheel : Inport  Port=2
  T_wheel : Inport  Port=3
  Constant : Constant  Value=gear_ratio
  Power flow : Subsystem
  Product : Product  SaturateOnIntegerOverflow=on  RndMeth=Zero  InputSameDT=on  OutDataTypeStr=Inherit: Same as first input
  Product1 : Product  SaturateOnIntegerOverflow=on  RndMeth=Zero  InputSameDT=on  OutDataTypeStr=Inherit: Same as first input
  Product3 : Product  SaturateOnIntegerOverflow=on  RndMeth=Zero  InputSameDT=on  OutDataTypeStr=Inherit: Same as first input
  To Workspace1 : ToWorkspace  VariableName=w_trans_2  SampleTime=-1
  To Workspace2 : ToWorkspace  VariableName=T_trans_2  SampleTime=-1
  To Workspace3 : ToWorkspace  VariableName=P_trans_2  SampleTime=-1
  w_trans : Outport  InitialOutput=0
  dw_trans : Outport  Port=2  InitialOutput=0
  T_trans : Outport  Port=3  InitialOutput=0
  wires:
  Product3/1 -> To Workspace3/1
  w_wheel/1 -> Power flow/1(w_wheel), Product/1
  Constant/1 -> Product/2, Product1/2, Power flow/3(gear_ratio)
  T_wheel/1 -> Power flow/2(T_wheel)
  dw_wheel/1 -> Product1/1
  Product/1 -> Product3/1, To Workspace1/1, w_trans/1
  Product1/1 -> dw_trans/1
  Power flow/1(T_trans) -> Product3/2, To Workspace2/1, T_trans/1

== system qss_tb_library_aalto/Gear System/Transmission CE-EG v2 ==
  w_CE : Inport
  dw_CE : Inport  Port=2
  T_CE : Inport  Port=3
  Constant : Constant  Value=gear_ratio
  Power flow : Subsystem
  Product : Product  SaturateOnIntegerOverflow=on  RndMeth=Zero  InputSameDT=on  OutDataTypeStr=Inherit: Same as first input
  Product1 : Product  SaturateOnIntegerOverflow=on  RndMeth=Zero  InputSameDT=on  OutDataTypeStr=Inherit: Same as first input
  Product3 : Product  SaturateOnIntegerOverflow=on  RndMeth=Zero  InputSameDT=on  OutDataTypeStr=Inherit: Same as first input
  To Workspace1 : ToWorkspace  VariableName=w_trans_2  SampleTime=-1
  To Workspace2 : ToWorkspace  VariableName=T_trans_2  SampleTime=-1
  To Workspace3 : ToWorkspace  VariableName=P_trans_2  SampleTime=-1
  w_trans : Outport  InitialOutput=0
  dw_trans : Outport  Port=2  InitialOutput=0
  T_trans : Outport  Port=3  InitialOutput=0
  wires:
  Power flow/1(T_trans) -> T_trans/1, To Workspace2/1, Product3/2
  Product1/1 -> dw_trans/1
  Product/1 -> w_trans/1, To Workspace1/1, Product3/1
  dw_CE/1 -> Product1/1
  T_CE/1 -> Power flow/2(T_wheel)
  Constant/1 -> Power flow/3(gear_ratio), Product1/2, Product/2
  w_CE/1 -> Product/1, Power flow/1(w_wheel)
  Product3/1 -> To Workspace3/1

== system qss_tb_library_aalto/Gear System/Transmission Vehicle-EM ==
  w_wheel : Inport
  dw_wheel : Inport  Port=2
  T_wheel : Inport  Port=3
  Constant : Constant  Value=gear_ratio
  Power flow : Subsystem
  Product : Product  SaturateOnIntegerOverflow=on  RndMeth=Zero  InputSameDT=on  OutDataTypeStr=Inherit: Same as first input
  Product1 : Product  SaturateOnIntegerOverflow=on  RndMeth=Zero  InputSameDT=on  OutDataTypeStr=Inherit: Same as first input
  Product3 : Product  SaturateOnIntegerOverflow=on  RndMeth=Zero  InputSameDT=on  OutDataTypeStr=Inherit: Same as first input
  To Workspace1 : ToWorkspace  VariableName=w_trans_1  SampleTime=-1
  To Workspace2 : ToWorkspace  VariableName=T_trans_1  SampleTime=-1
  To Workspace3 : ToWorkspace  VariableName=P_trans_1  SampleTime=-1
  w_trans : Outport  InitialOutput=0
  dw_trans : Outport  Port=2  InitialOutput=0
  T_trans : Outport  Port=3  InitialOutput=0
  wires:
  Product3/1 -> To Workspace3/1
  w_wheel/1 -> Power flow/1(w_wheel), Product/1
  Constant/1 -> Product/2, Product1/2, Power flow/3(gear_ratio)
  T_wheel/1 -> Power flow/2(T_wheel)
  dw_wheel/1 -> Product1/1
  Product/1 -> Product3/1, To Workspace1/1, w_trans/1
  Product1/1 -> dw_trans/1
  Power flow/1(T_trans) -> Product3/2, To Workspace2/1, T_trans/1

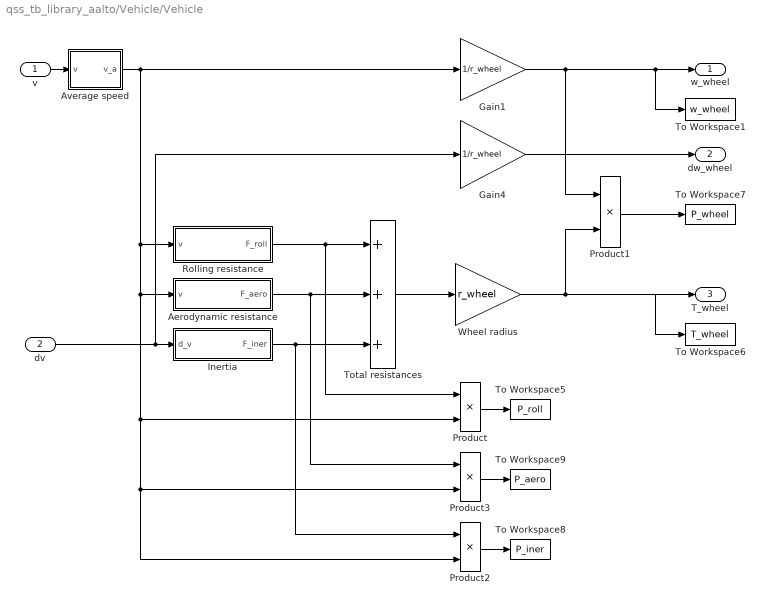
== system qss_tb_library_aalto/Vehicle/Vehicle ==
  v : Inport
  dv : Inport  Port=2
  Aerodynamic resistance : Subsystem
  Average speed : Subsystem
  Gain1 : Gain  Gain=1/r_wheel  SaturateOnIntegerOverflow=on  OutDataTypeStr=Inherit: Same as input  ParamDataTypeStr=Inherit: Same as input
  Gain4 : Gain  Gain=1/r_wheel  SaturateOnIntegerOverflow=on  OutDataTypeStr=Inherit: Same as input  ParamDataTypeStr=Inherit: Same as input
  Inertia : Subsystem
  Product{,1..3} (4 alike) : Product  SaturateOnIntegerOverflow=on  RndMeth=Zero  InputSameDT=on  OutDataTypeStr=Inherit: Same as first input
  Rolling resistance : Subsystem
  To Workspace1 : ToWorkspace  VariableName=w_wheel  SampleTime=-1
  To Workspace5 : ToWorkspace  VariableName=P_roll  SampleTime=-1
  To Workspace6 : ToWorkspace  VariableName=T_wheel  SampleTime=-1
  To Workspace7 : ToWorkspace  VariableName=P_wheel  SampleTime=-1
  To Workspace8 : ToWorkspace  VariableName=P_iner  SampleTime=-1
  To Workspace9 : ToWorkspace  VariableName=P_aero  SampleTime=-1
  Total resistances : Sum  Inputs=+++  SaturateOnIntegerOverflow=on  InputSameDT=on  OutDataTypeStr=Inherit: Same as first input
  Wheel radius : Gain  Gain=r_wheel  SaturateOnIntegerOverflow=on  OutDataTypeStr=Inherit: Same as input  ParamDataTypeStr=Inherit: Same as input
  w_wheel : Outport  InitialOutput=0
  dw_wheel : Outport  Port=2  InitialOutput=0
  T_wheel : Outport  Port=3  InitialOutput=0
  wires:
  Gain4/1 -> dw_wheel/1
  Gain1/1 -> Product1/1, w_wheel/1, To Workspace1/1
  Rolling resistance/1(F_roll) -> Total resistances/1, Product/1
  Aerodynamic resistance/1(F_aero) -> Product3/1, Total resistances/2
  Inertia/1(F_iner) -> Total resistances/3, Product2/1
  Total resistances/1 -> Wheel radius/1
  Wheel radius/1 -> T_wheel/1, Product1/2, To Workspace6/1
  Average speed/1(v_a) -> Gain1/1, Aerodynamic resistance/1(v), Product/2, Product3/2, Product2/2, Rolling resistance/1(v)
  dv/1 -> Inertia/1(d_v), Gain4/1
  v/1 -> Average speed/1(v)
  Product2/1 -> To Workspace8/1
  Product3/1 -> To Workspace9/1
  Product1/1 -> To Workspace7/1
  Product/1 -> To Workspace5/1

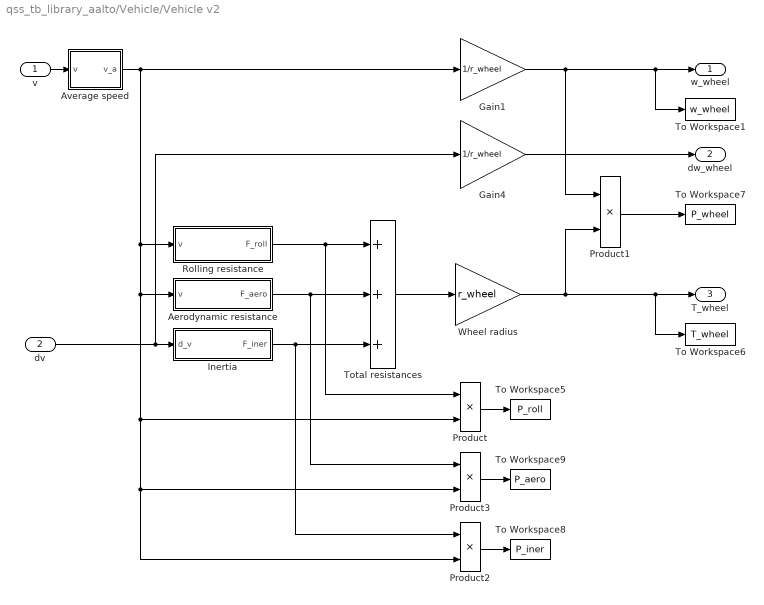
== system qss_tb_library_aalto/Vehicle/Vehicle v2 ==
  v : Inport
  dv : Inport  Port=2
  Aerodynamic resistance : Subsystem
  Average speed : Subsystem
  Gain1 : Gain  Gain=1/r_wheel  SaturateOnIntegerOverflow=on  OutDataTypeStr=Inherit: Same as input  ParamDataTypeStr=Inherit: Same as input
  Gain4 : Gain  Gain=1/r_wheel  SaturateOnIntegerOverflow=on  OutDataTypeStr=Inherit: Same as input  ParamDataTypeStr=Inherit: Same as input
  Inertia : Subsystem
  Product{,1..3} (4 alike) : Product  SaturateOnIntegerOverflow=on  RndMeth=Zero  InputSameDT=on  OutDataTypeStr=Inherit: Same as first input
  Rolling resistance : Subsystem
  To Workspace1 : ToWorkspace  VariableName=w_wheel  SampleTime=-1
  To Workspace5 : ToWorkspace  VariableName=P_roll  SampleTime=-1
  To Workspace6 : ToWorkspace  VariableName=T_wheel  SampleTime=-1
  To Workspace7 : ToWorkspace  VariableName=P_wheel  SampleTime=-1
  To Workspace8 : ToWorkspace  VariableName=P_iner  SampleTime=-1
  To Workspace9 : ToWorkspace  VariableName=P_aero  SampleTime=-1
  Total resistances : Sum  Inputs=+++  SaturateOnIntegerOverflow=on  InputSameDT=on  OutDataTypeStr=Inherit: Same as first input
  Wheel radius : Gain  Gain=r_wheel  SaturateOnIntegerOverflow=on  OutDataTypeStr=Inherit: Same as input  ParamDataTypeStr=Inherit: Same as input
  w_wheel : Outport  InitialOutput=0
  dw_wheel : Outport  Port=2  InitialOutput=0
  T_wheel : Outport  Port=3  InitialOutput=0
  wires:
  Product/1 -> To Workspace5/1
  Product1/1 -> To Workspace7/1
  Product3/1 -> To Workspace9/1
  Product2/1 -> To Workspace8/1
  v/1 -> Average speed/1(v)
  dv/1 -> Gain4/1, Inertia/1(d_v)
  Average speed/1(v_a) -> Rolling resistance/1(v), Product2/2, Product3/2, Product/2, Aerodynamic resistance/1(v), Gain1/1
  Wheel radius/1 -> To Workspace6/1, T_wheel/1, Product1/2
  Total resistances/1 -> Wheel radius/1
  Inertia/1(F_iner) -> Product2/1, Total resistances/3
  Aerodynamic resistance/1(F_aero) -> Total resistances/2, Product3/1
  Rolling resistance/1(F_roll) -> Product/1, Total resistances/1
  Gain1/1 -> To Workspace1/1, w_wheel/1, Product1/1
  Gain4/1 -> dw_wheel/1

== system qss_tb_library_aalto/Controller/Battery Controller/Geno-Group On ==
  cc_on : Inport
  Clock : Subsystem  mask(Digital clock){}
      mask help:
      | Digital clock.
      | Output is set to 1 for the first half of the period.
      mask init:
      | duration = @1/2;
      mask Help: Digital clock for logic systems.
      mask Display: plot(0,0,100,100,[90,75,75,60,60,35,35,20,20,10],[20,20,80,80,19,20,80,80,20,20])
  Constant : Constant  Value=cc_done
  Counter : UnitDelay  SampleTime=h
  Data Type Conversion1 : DataTypeConversion  OutDataTypeStr=boolean
  Data Type Conversion2 : DataTypeConversion  OutDataTypeStr=double
  Data Type Conversion3 : DataTypeConversion  OutDataTypeStr=double
  Logical operator3 : Logic
  Mux : Mux  Inputs=3
  Product : Product  SaturateOnIntegerOverflow=on  RndMeth=Zero  InputSameDT=on  OutDataTypeStr=Inherit: Same as first input
  Relational Operator : RelationalOperator  OutDataTypeStr=boolean  InputSameDT=on
  Sum3 : Sum  Inputs=++-  SaturateOnIntegerOverflow=on  InputSameDT=on  OutDataTypeStr=Inherit: Same as first input
  T_EG start-up : Lookup  InputValues=t_c  Table=T_EG_c  SaturateOnIntegerOverflow=on
  dw start-up : Lookup  InputValues=t_c  Table=dw_GG_c  SaturateOnIntegerOverflow=on
  w start-up : Lookup  InputValues=t_c  Table=w_GG_c  SaturateOnIntegerOverflow=on
  OutOn : Outport  InitialOutput=0
  done : Outport  Port=2  InitialOutput=0
  wires:
  Data Type Conversion3/1 -> Product/1
  Data Type Conversion2/1 -> Sum3/2
  Data Type Conversion1/1 -> Logical operator3/2
  Mux/1 -> OutOn/1
  T_EG start-up/1 -> Mux/3
  dw start-up/1 -> Mux/2
  w start-up/1 -> Mux/1
  Logical operator3/1 -> Data Type Conversion2/1
  Counter/1 -> Sum3/1, dw start-up/1, T_EG start-up/1, Product/2, Relational Operator/1, w start-up/1
  Sum3/1 -> Counter/1
  Clock/1(out_1) -> Data Type Conversion1/1
  cc_on/1 -> Logical operator3/1
  Product/1 -> Sum3/3
  Constant/1 -> Relational Operator/2
  Relational Operator/1 -> Data Type Conversion3/1, done/1

== system qss_tb_library_aalto/Controller/Battery Controller/S-R Flip-Flop ==
  S : Inport
  R : Inport  Port=2
  Demux : Demux  Outputs=2
  Logic : CombinatorialLogic  TruthTable=[0 1;0 1;1 0;0 1;1 0;0 1;1 0;1 0]
  Memory : Memory  InheritSampleTime=on
  Mux : Mux  Inputs=3
  Q : Outport  InitialOutput=0
  !Q : Outport  Port=2  InitialOutput=1
  wires:
  R/1 -> Mux/3
  S/1 -> Mux/2
  Memory/1 -> Mux/1
  Demux/1 -> Memory/1, Q/1
  Demux/2 -> !Q/1
  Logic/1 -> Demux/1
  Mux/1 -> Logic/1

== system qss_tb_library_aalto/Controller/Gen-set Controller v2/Engine start control ==
  speed (m/s) : Inport
  soc : Inport  Port=2
  Constant11 : Constant  Value=10  OutDataTypeStr=double
  Cst_Q_BT_max : Constant  Value=soc_max
  Cst_Q_BT_min : Constant  Value=soc_min
  Data Type Conversion2 : DataTypeConversion  OutDataTypeStr=double
  Engine on off : Subsystem
  Hit Crossing : HitCross  HitCrossingOffset=0.5  HitCrossingDirection=rising
  Logical operator1 : Logic  Operator=OR
  Logical operator2 : Logic  Operator=OR
  Logical operator3 : Logic  Operator=OR
  Relational Operator : RelationalOperator  Operator=<=  OutDataTypeStr=boolean
  Relational Operator1 : RelationalOperator  OutDataTypeStr=boolean
  Terminator2 : Terminator
  low speed : simulink/Logic and Bit Operations/Compare To Constant  relop=<=  const=1  OutDataTypeStr=boolean
  speed min-max : Relay  OnSwitchValue=spd_max/3.6  OffSwitchValue=spd_min/3.6  OutDataTypeStr=Inherit: Inherit via back propagation
  tempo : Subsystem
      mask Display: disp('Tempo')
  engine on : Outport
  wires:
  speed min-max/1 -> Logical operator3/1
  low speed/1 -> Logical operator1/1
  Logical operator2/1 -> engine on/1
  tempo/1(tempo) -> Logical operator2/2
  Data Type Conversion2/1 -> Logical operator2/1, Hit Crossing/1
  Engine on off/1(Q) -> Data Type Conversion2/1
  Hit Crossing/1 -> tempo/1(flag)
  Constant11/1 -> tempo/2(time)
  Relational Operator1/1 -> Logical operator1/2
  soc/1 -> Relational Operator1/1, Relational Operator/1
  Engine on off/2(!Q) -> Terminator2/1
  Logical operator1/1 -> Engine on off/2(R)
  Logical operator3/1 -> Engine on off/1(S)
  speed (m/s)/1 -> low speed/1, speed min-max/1
  Cst_Q_BT_max/1 -> Relational Operator1/2
  Relational Operator/1 -> Logical operator3/2
  Cst_Q_BT_min/1 -> Relational Operator/2

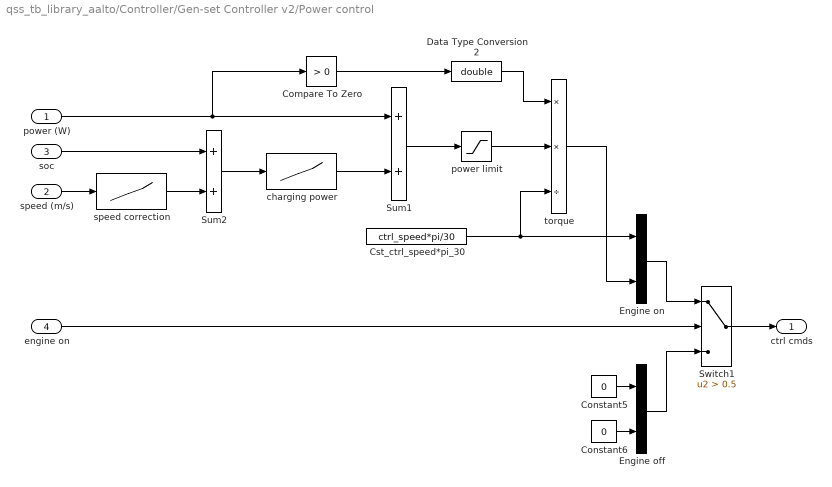
== system qss_tb_library_aalto/Controller/Gen-set Controller v2/Power control ==
  power (W) : Inport
  speed (m/s) : Inport  Port=2
  soc : Inport  Port=3
  engine on : Inport  Port=4
  Compare To Zero : simulink/Logic and Bit Operations/Compare To Zero  relop=>  OutDataTypeStr=boolean
  Constant5 : Constant  Value=0  OutDataTypeStr=double
  Constant6 : Constant  Value=0  OutDataTypeStr=double
  Cst_ctrl_speed*pi_30 : Constant  Value=ctrl_speed*pi/30  OutDataTypeStr=double  SampleTime=Inf
  Data Type Conversion2 : DataTypeConversion  OutDataTypeStr=double
  Engine off : Mux  Inputs=2
  Engine on : Mux  Inputs=2
  Sum1 : Sum  SaturateOnIntegerOverflow=on  InputSameDT=on  OutDataTypeStr=Inherit: Same as first input
  Sum2 : Sum  SaturateOnIntegerOverflow=on  InputSameDT=on  OutDataTypeStr=Inherit: Same as first input
  Switch1 : Switch  Criteria=u2 > Threshold  Threshold=0.5  SaturateOnIntegerOverflow=on  InputSameDT=on
  charging power : Lookup_n-D  NumberOfTableDimensions=1  BreakpointsForDimension1=[0 0.6 0.71 0.75 0.8 1]  Table=[power_max power_max 0 0 -power_max/2 -power_max/2]  RndMeth=Simplest  InputSameDT=on
  power limit : Saturate  UpperLimit=power_max  LowerLimit=0
  speed correction : Lookup_n-D  NumberOfTableDimensions=1  BreakpointsForDimension1=[0 120]/3.6  Table=[0 spd_coeff]  RndMeth=Simplest  InputSameDT=on
  torque : Product  Inputs=**/  SaturateOnIntegerOverflow=on  RndMeth=Zero  InputSameDT=on  OutDataTypeStr=Inherit: Same as first input
  ctrl cmds : Outport
  wires:
  speed correction/1 -> Sum2/2
  power (W)/1 -> Sum1/1, Compare To Zero/1
  charging power/1 -> Sum1/2
  Sum2/1 -> charging power/1
  soc/1 -> Sum2/1
  speed (m/s)/1 -> speed correction/1
  Switch1/1 -> ctrl cmds/1
  engine on/1 -> Switch1/2
  Cst_ctrl_speed*pi_30/1 -> torque/3, Engine on/1
  torque/1 -> Engine on/2
  Sum1/1 -> power limit/1
  Engine off/1 -> Switch1/3
  Engine on/1 -> Switch1/1
  Constant6/1 -> Engine off/2
  Constant5/1 -> Engine off/1
  power limit/1 -> torque/2
  Compare To Zero/1 -> Data Type Conversion2/1
  Data Type Conversion2/1 -> torque/1
